simulink model "duffing"  (R2020a)
settings: Solver=VariableStepAuto  StartTime=0.0  StopTime=10.0  RelTol=1e-3
undefined symbols (not defined in the file or in its folder): alpha, duffing_func, g, k, l, linsys, m, x_init_NL
settings Model: Creator=jbrouill  LastModifiedBy=clara
settings DataIOCC: Refine=10

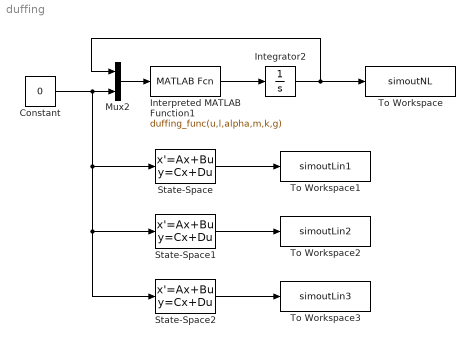
== system duffing ==
  Constant : Constant  Value=0
  Integrator2 : Integrator  InitialCondition=x_init_NL
  Interpreted MATLAB Function1 : MATLABFcn  MATLABFcn=duffing_func(u,l,alpha,m,k,g)
  Mux2 : Mux  Inputs=2
  State-Space : StateSpace  A=linsys(1).A  B=linsys(1).B  C=linsys(1).C  D=linsys(1).D  InitialCondition=linsys(1).x_init
  State-Space1 : StateSpace  A=linsys(2).A  B=linsys(2).B  C=linsys(2).C  D=linsys(2).D  InitialCondition=linsys(2).x_init
  State-Space2 : StateSpace  A=linsys(3).A  B=linsys(3).B  C=linsys(3).C  D=linsys(3).D  InitialCondition=linsys(3).x_init
  To Workspace : ToWorkspace  VariableName=simoutNL  SampleTime=-1
  To Workspace1 : ToWorkspace  VariableName=simoutLin1  SampleTime=-1
  To Workspace2 : ToWorkspace  VariableName=simoutLin2  SampleTime=-1
  To Workspace3 : ToWorkspace  VariableName=simoutLin3  SampleTime=-1
  wires:
  Constant/1 -> State-Space2/1, State-Space1/1, State-Space/1, Mux2/2
  State-Space/1 -> To Workspace1/1
  State-Space1/1 -> To Workspace2/1
  State-Space2/1 -> To Workspace3/1
  Mux2/1 -> Interpreted MATLAB Function1/1
  Integrator2/1 -> To Workspace/1, Mux2/1
  Interpreted MATLAB Function1/1 -> Integrator2/1
